simulink model "model"  (R2020a)
settings: Solver=VariableStepAuto  StartTime=0.0  StopTime=10.0  RelTol=1e-3
settings Model: Creator=PRATIKSHA  LastModifiedBy=PRATIKSHA

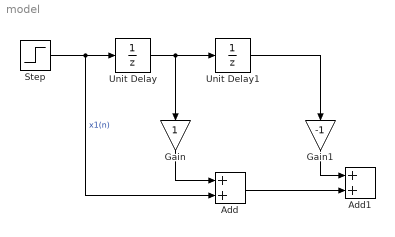
== system model ==
  Add : Sum
  Add1 : Sum
  Gain : Gain
  Gain1 : Gain  Gain=-1
  Step : Step  SampleTime=0
  Unit Delay : UnitDelay  SampleTime=-1  HasFrameUpgradeWarning=on
  Unit Delay1 : UnitDelay  SampleTime=-1  HasFrameUpgradeWarning=on
  wires:
  Unit Delay/1 -> Gain/1, Unit Delay1/1
  Gain/1 -> Add/1
  Step/1 -> Add/2, Unit Delay/1  "x1(n)"
  Gain1/1 -> Add1/1
  Unit Delay1/1 -> Gain1/1
  Add/1 -> Add1/2
